simulink model "cascadeControl"  (R2020a)
settings: Solver=VariableStepAuto  StartTime=0.0  StopTime=40.0  RelTol=1e-3
values from neighbouring files (symbols this model uses):
  condtheta = 0.2    [initialization.m]
  condx = 1    [initialization.m]
  condy = 0    [initialization.m]
  k = 10    [initialization.m]
  k_omega = 1    [initialization.m]
settings Model: Creator=adelina  LastModifiedBy=adelina

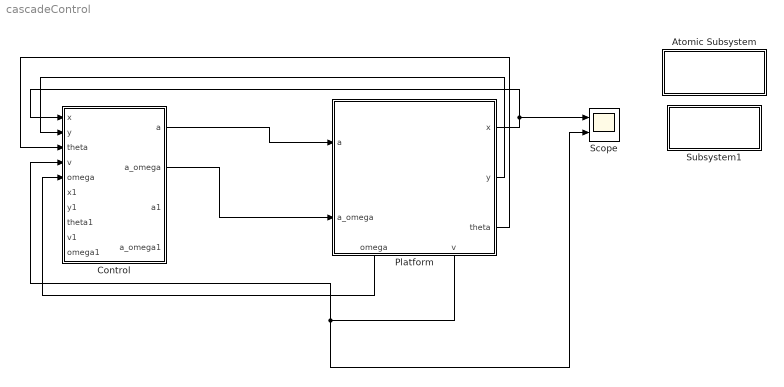
== system cascadeControl ==
  Atomic Subsystem : Subsystem  TreatAsAtomicUnit=on
      settings: OpenFcn=initialization
      mask Display: disp('initialization')
  Control : Subsystem
  Platform : Subsystem
      settings: PortSchema="{\"entries\":[{\"content\":{\"sides\":[{\"content\":{\"connectorIds\":[\"In1\",\"In2\"]},\"type\":\"ConnectorPlacement.EquallySpacedRectSide\",\"uuid\":\"a1c86654-af40-4ad6-a974-25f87faec7d4\"},{\"content\":{\"connectorIds\":[\"Out1\",\"Out2\",\"Out3\"],\"side\":\"RIGHT\"},\"type\":\"ConnectorPlacement.EquallySpacedRectSide\",\"uuid\":\"7d2d01bc-12a9-4b94-952e-ee76a503b378\"},{\"content\":{\"connectorIds\":[],\"side\":\"TOP\"},\"type\":\"ConnectorPlacement.EquallySpacedRectSide\",\"uuid\":\"d40a5efb-aa90-45b2-a018-62ed5e210de3\"},{\"content\":{\"connectorIds\":[\"Out4\",\"Out5\"],\"side\":\"BOTTOM\"},\"type\":\"ConnectorPlacement.EquallySpacedRectSide\",\"uuid\":\"3a1daf5d-2eda-4580-9484-1f68c5a9e1d3\"}]},\"type\":\"ConnectorPlacement.EquallySpacedConnector\",\"uuid\":\"38cf7c1a-3443-4b69-bcc1-3393400aa111\"}],\"packageUris\":[\"http://schema.mathworks.com/mf0/Connector/19700101\"],\"version\":\"1.0\"}"
  Scope : Scope  NumInputPorts=2
  Subsystem1 : Subsystem
      settings: OpenFcn=plots
      mask Display: disp('plots')
  wires:
  Control/1(a) -> Platform/1(a)
  Control/2(a_omega) -> Platform/2(a_omega)
  Platform/1(x) -> Scope/1, Control/1(x)
  Platform/2(y) -> Control/2(y)
  Platform/3(theta) -> Control/3(theta)
  Platform/4(omega) -> Control/5(omega)
  Platform/5(v) -> Scope/2, Control/4(v)

== system cascadeControl/Atomic Subsystem ==

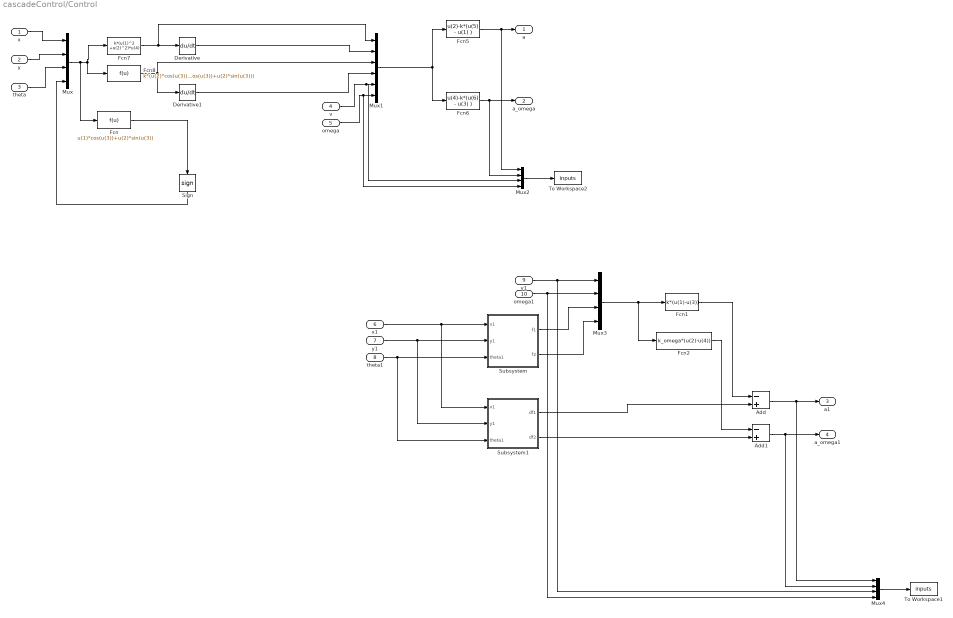
== system cascadeControl/Control ==
  x : Inport
  y : Inport  Port=2
  theta : Inport  Port=3
  v : Inport  Port=4
  omega : Inport  Port=5
  x1 : Inport  Port=6
  y1 : Inport  Port=7
  theta1 : Inport  Port=8
  v1 : Inport  Port=9
  omega1 : Inport  Port=10
  Add : Sum  Inputs=-+
  Add1 : Sum  Inputs=-+
  Derivative : Derivative
  Derivative1 : Derivative
  Fcn : Fcn  Expr=u(1)*cos(u(3))+u(2)*sin(u(3))
  Fcn1 : Fcn  Expr=k*(u(1)-u(3))
  Fcn2 : Fcn  Expr=k_omega*(u(2)-u(4))
  Fcn5 : Fcn  Expr=u(2)-k*(u(5) - u(1) )
  Fcn6 : Fcn  Expr=u(4)-k*(u(6) - u(3) )
  Fcn7 : Fcn  Expr=k*(u(1)^2 +u(2)^2)*u(4)
  Fcn8 : Fcn  Expr=k*(u(2)*cos(u(3))-u(1)*sin(u(3)))*(u(1)*cos(u(3))+u(2)*sin(u(3)))
  Mux{,2..4} (4 alike) : Mux
  Mux1 : Mux  Inputs=6
  Sign : Signum
  Subsystem : Subsystem
  Subsystem1 : Subsystem
  To Workspace1 : ToWorkspace  VariableName=inputs  SaveFormat=Structure With Time  SampleTime=-1
  To Workspace2 : ToWorkspace  VariableName=inputs  SaveFormat=Structure With Time  SampleTime=-1
  a : Outport
  a_omega : Outport  Port=2
  a1 : Outport  Port=3
  a_omega1 : Outport  Port=4
  wires:
  Fcn6/1 -> Mux2/2, a_omega/1
  Fcn7/1 -> Mux1/1, Derivative/1
  Mux1/1 -> Fcn5/1, Fcn6/1
  Mux2/1 -> To Workspace2/1
  Fcn5/1 -> Mux2/1, a/1
  x/1 -> Mux/1
  y/1 -> Mux/2
  theta/1 -> Mux/3
  Mux/1 -> Fcn7/1, Fcn8/1, Fcn/1
  Fcn8/1 -> Derivative1/1, Mux1/3
  Derivative/1 -> Mux1/2
  Derivative1/1 -> Mux1/4
  v/1 -> Mux2/3, Mux1/5
  omega/1 -> Mux2/4, Mux1/6
  Fcn/1 -> Sign/1
  Sign/1 -> Mux/4
  x1/1 -> Subsystem1/1(x1), Subsystem/1(x1)
  y1/1 -> Subsystem1/2(y1), Subsystem/2(y1)
  theta1/1 -> Subsystem1/3(theta1), Subsystem/3(theta1)
  Subsystem/1(f1) -> Mux3/3
  Subsystem/2(f2) -> Mux3/4
  Mux3/1 -> Fcn2/1, Fcn1/1
  Subsystem1/1(df1) -> Add/2
  Fcn1/1 -> Add/1
  Fcn2/1 -> Add1/1
  Subsystem1/2(df2) -> Add1/2
  v1/1 -> Mux4/3, Mux3/1
  Mux4/1 -> To Workspace1/1
  Add1/1 -> Mux4/2, a_omega1/1
  Add/1 -> Mux4/1, a1/1
  omega1/1 -> Mux4/4, Mux3/2

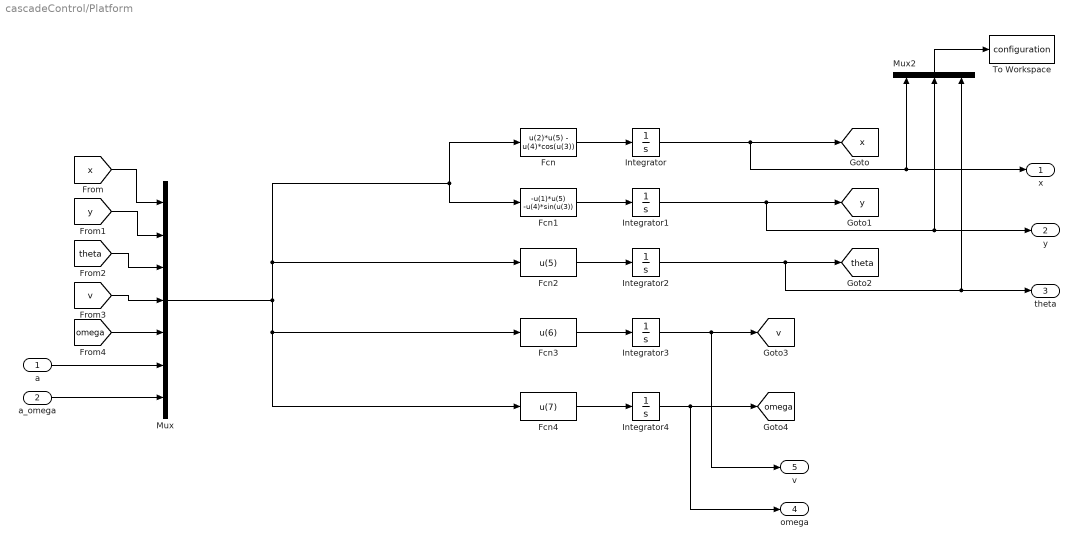
== system cascadeControl/Platform ==
  a : Inport
  a_omega : Inport  Port=2
  Fcn : Fcn  Expr=u(2)*u(5) - u(4)*cos(u(3))
  Fcn1 : Fcn  Expr=-u(1)*u(5) -u(4)*sin(u(3))
  Fcn2 : Fcn  Expr=u(5)
  Fcn3 : Fcn  Expr=u(6)
  Fcn4 : Fcn  Expr=u(7)
  Integrator : Integrator  InitialCondition=condx
  Integrator1 : Integrator  InitialCondition=condy
  Integrator2 : Integrator  InitialCondition=condtheta
  Integrator3 : Integrator
  Integrator4 : Integrator
  Mux : Mux  Inputs=7
  Mux2 : Mux  Inputs=3
  To Workspace : ToWorkspace  VariableName=configuration  SaveFormat=Structure With Time  SampleTime=-1
  x : Outport
  y : Outport  Port=2
  theta : Outport  Port=3
  omega : Outport  Port=4
  v : Outport  Port=5
  tag scope: omega=global, theta=global, v=global, x=global, y=global
  wires:
  Fcn2/1 -> Integrator2/1
  Integrator3/1 -> v/1, [v]
  [v] -> Mux/4
  Integrator2/1 -> theta/1, Mux2/3, [theta]
  [omega] -> Mux/5
  Fcn3/1 -> Integrator3/1
  Fcn1/1 -> Integrator1/1
  [y] -> Mux/2
  Integrator4/1 -> omega/1, [omega]
  [x] -> Mux/1
  Fcn4/1 -> Integrator4/1
  a/1 -> Mux/6
  Mux/1 -> Fcn1/1, Fcn/1, Fcn2/1, Fcn4/1, Fcn3/1
  Integrator1/1 -> y/1, Mux2/2, [y]
  [theta] -> Mux/3
  Integrator/1 -> x/1, Mux2/1, [x]
  Fcn/1 -> Integrator/1
  a_omega/1 -> Mux/7
  Mux2/1 -> To Workspace/1

== system cascadeControl/Subsystem1 ==

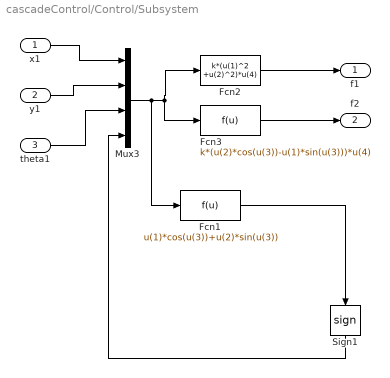
== system cascadeControl/Control/Subsystem ==
  x1 : Inport
  y1 : Inport  Port=2
  theta1 : Inport  Port=3
  Fcn1 : Fcn  Expr=u(1)*cos(u(3))+u(2)*sin(u(3))
  Fcn2 : Fcn  Expr=k*(u(1)^2 +u(2)^2)*u(4)
  Fcn3 : Fcn  Expr=k*(u(2)*cos(u(3))-u(1)*sin(u(3)))*u(4)
  Mux3 : Mux
  Sign1 : Signum
  f1 : Outport
  f2 : Outport  Port=2
  wires:
  Sign1/1 -> Mux3/4
  y1/1 -> Mux3/2
  x1/1 -> Mux3/1
  theta1/1 -> Mux3/3
  Fcn1/1 -> Sign1/1
  Mux3/1 -> Fcn2/1, Fcn3/1, Fcn1/1
  Fcn2/1 -> f1/1
  Fcn3/1 -> f2/1

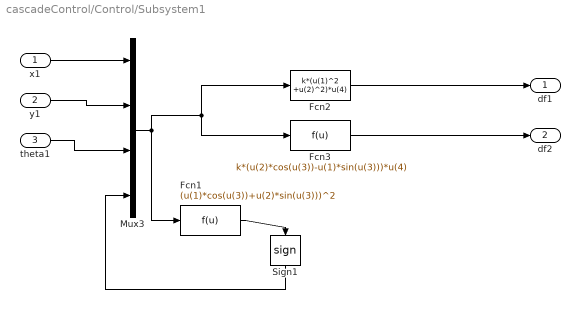
== system cascadeControl/Control/Subsystem1 ==
  x1 : Inport
  y1 : Inport  Port=2
  theta1 : Inport  Port=3
  Fcn1 : Fcn  Expr=(u(1)*cos(u(3))+u(2)*sin(u(3)))^2
  Fcn2 : Fcn  Expr=k*(u(1)^2 +u(2)^2)*u(4)
  Fcn3 : Fcn  Expr=k*(u(2)*cos(u(3))-u(1)*sin(u(3)))*u(4)
  Mux3 : Mux
  Sign1 : Signum
  df1 : Outport
  df2 : Outport  Port=2
  wires:
  Sign1/1 -> Mux3/4
  y1/1 -> Mux3/2
  x1/1 -> Mux3/1
  theta1/1 -> Mux3/3
  Fcn1/1 -> Sign1/1
  Mux3/1 -> Fcn2/1, Fcn3/1, Fcn1/1
  Fcn2/1 -> df1/1
  Fcn3/1 -> df2/1
